simulink model "controlador_trebol"  (R2025b)
settings: Solver=FixedStepDiscrete  StartTime=0.0  StopTime=inf  FixedStep=0.1  RelTol=1e-3
settings Model: Creator=isaac-silias  LastModifiedBy=saumnty

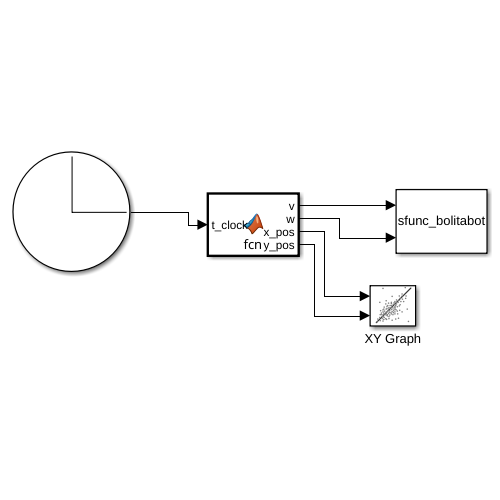
[thumbnail: Simulink's stored preview of the top-level diagram]
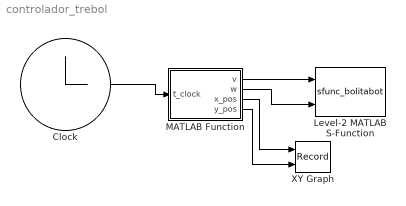
== system controlador_trebol ==
  Clock : Clock
  Level-2 MATLAB S-Function : M-S-Function  FunctionName=sfunc_bolitabot
  MATLAB Function : MATLAB Function  TreatAsAtomicUnit=on
  XY Graph : Record  NumPorts=2.0  FileSettingsInternal="{\"entries\":[{\"content\":{\"excelSettings\":{\"content\":{},\"type\":\"Streamout.ExcelSettings\"},\"parquetSettings\":{\"content\":{},\"type\":\"Streamout.ParquetSettings\"}},\"type\":\"Streamout.FileSettingStorage\",\"uuid\":\"\"}],\"packageUris\":[\"http:\\/\\/schema.mathworks.com\\/mf0\\/streamout_blocks\\/R2020a\"],\"version\":\"1.0\"}"  FrameSettings=[0, 0]  Layout=[1 1]  SignalsInternal="{\"entries\":[{\"content\":{\"signals\":[{\"content\":{\"blockPath\":[],\"dimensions\":[1],\"domain\":\"\",\"lineColor\":\"#a2142f\",\"plots\":[ 1 ],\"port\":1,\"sid\":[\"\"],\"signalID\":1,\"signalName\":\"MATLAB Function:3\"},\"type\":\"RecordBlkView.Signal\",\"uuid\":\"\"},{\"content\":{\"blockPath\":[],\"dimensions\":[1],\"domain\":\"\",\"lineColor\":\"#139fff\",\"plots\":[ 1 ],\"port\":2,\"sid\":[\"\"],\"signalID\":2,\"signalName\":\"MATLAB Function:4\"},\"type\":\"RecordBlkView.Signal\",\"uuid\":\"\"}]},\"type\":\"RecordBlkView.InputSignals\",\"uuid\":\"\"}],\"packageUris\":[\"http:\\/\\/schema.mathworks.com\\/mf0\\/streamout_blocks\\/R2020a\"],\"version\":\"1.0\"}"  VisualizationBindings="{\"xyplotplugin\":{\"info\":[{\"series\":[{\"bindingParametersList\":[{\"parameter\":\"X-Axis\",\"signalID\":1,\"signalName\":\"MATLAB Function:3\"},{\"parameter\":\"Y-Axis\",\"signalID\":2,\"signalName\":\"MATLAB Function:4\"}],\"seriesID\":0}],\"subplotID\":1}]}}"  CompatibilityTag=XY
  wires:
  Clock/1 -> MATLAB Function/1(t_clock)
  MATLAB Function/3(x_pos) -> XY Graph/1
  MATLAB Function/4(y_pos) -> XY Graph/2
  MATLAB Function/1(v) -> Level-2 MATLAB S-Function/1
  MATLAB Function/2(w) -> Level-2 MATLAB S-Function/2

== matlab function controlador_trebol/MATLAB Function ==
  data: t_clock input; v output; w output; x_pos output; y_pos output
function [v, w, x_pos, y_pos] = fcn(t_clock)
    coder.extrinsic('py.brain_hermite.get_hermite_point');
    coder.extrinsic('leer_odom');
    coder.extrinsic('get_tramo');

    v=0.0; w=0.0; x_pos=0.0; y_pos=0.0;
    P0=[0.0,0.0]; P1=[0.0,0.0];
    V0=[0.0,0.0]; V1=[0.0,0.0];
    t_hermite=0.0; tramo=0; T_actual=6.0;
    encontrado=0; temp_sum=0.0;
    x_r=0.0; y_r=0.0; theta_r=0.0;
    vx_h=0.0; vy_h=0.0;
    x_front=0.0; y_front=0.0;
    ex=0.0; ey=0.0; ux=0.0; uy=0.0;

    % --- TIEMPOS: 16 tramos (trebol simplificado) ---
    T_v = [6.0,6.0,6.0,6.0, ...
           6.0,6.0,6.0,6.0, ...
           6.0,6.0,6.0,6.0, ...
           6.0,6.0,6.0,6.0];

    t_total_ciclo = sum(T_v);
    t_relativo = mod(t_clock, t_total_ciclo);

    % --- BÚSQUEDA DE TRAMO ---
    for i = 1:length(T_v)
        if (encontrado==0) && (t_relativo < (temp_sum + T_v(i)))
            tramo = i-1;
            t_hermite = (t_relativo - temp_sum) / T_v(i);
            T_actual = T_v(i);
            encontrado = 1;
        end
        if encontrado==0
            temp_sum = temp_sum + T_v(i);
        end
    end

    % --- PUNTOS DE CONTROL ---
    [P0, P1, V0, V1] = get_tramo(tramo);
    P0=double(P0); P1=double(P1);
    V0=double(V0); V1=double(V1);

    % --- HERMITE ---
    p0_py={double(P0(1)),double(P0(2))};
    p1_py={double(P1(1)),double(P1(2))};
    v0_py={double(V0(1)),double(V0(2))};
    v1_py={double(V1(1)),double(V1(2))};

    res_py = py.brain_hermite.get_hermite_point( ...
        double(t_hermite), p0_py, p1_py, v0_py, v1_py);

    datos = zeros(1,6);
    datos = double(res_py);
    x_pos = double(datos(1));
    y_pos = double(datos(2));
    vx_h  = double(datos(3)) / T_actual;
    vy_h  = double(datos(4)) / T_actual;

    % --- ODOMETRÍA ---
    [x_r, y_r, theta_r] = leer_odom();
    x_r=double(x_r); y_r=double(y_r); theta_r=double(theta_r);

    % ============================================================
    % CONTROL DE PUNTO ADELANTADO (look-ahead point control)
    % ============================================================
    h = 0.5;
    Kx = 0.4;
    Ky = 0.5;
    v_max = 0.7;
    w_max = 1.0;

    x_front = x_r + h*cos(theta_r);
    y_front = y_r + h*sin(theta_r);

    ex = x_pos - x_front;
    ey = y_pos - y_front;

    ux = vx_h + Kx*ex;
    uy = vy_h + Ky*ey;

    v = cos(theta_r)*ux + sin(theta_r)*uy;
    w = (-sin(theta_r)*ux + cos(theta_r)*uy) / h;

    if v > v_max;  v = v_max;  end
    if v < -v_max; v = -v_max; end
    if w > w_max;  w = w_max;  end
    if w < -w_max; w = -w_max; end

    % ============================================================
    % CONTROL ANTERIOR (lazo cerrado clásico) — COMENTADO
    % ============================================================
    %{
    dist = sqrt(ex*ex + ey*ey);
    speed_h = sqrt(vx_h*vx_h + vy_h*vy_h);
    if dist > 1.5
        theta_d = atan2(ey, ex);
    else
        if speed_h > 0.001
            theta_d = atan2(vy_h, vx_h);
        else
            theta_d = atan2(ey, ex);
        end
    end
    e_theta = theta_d - theta_r;
    while e_theta > 3.14159;  e_theta = e_theta - 2.0*3.14159; end
    while e_theta < -3.14159; e_theta = e_theta + 2.0*3.14159; end
    Kv = 0.35; Kw = 1.2;
    v_max_old = 0.6;
    if abs(e_theta) > 0.3
        v = 0.0; w = Kw * e_theta;
    elseif abs(e_theta) > 0.1
        v = 0.1; w = Kw * e_theta;
    elseif dist > 1.5
        v = Kv * dist; w = Kw * e_theta;
    else
        v = 0.3; w = Kw * e_theta;
    end
    if v > v_max_old; v = v_max_old; end
    if v < 0.0;        v = 0.0;       end
    if w > 1.2;        w = 1.2;       end
    if w < -1.2;       w = -1.2;      end
    %}
end
